simulink subsystem "throttleInput"  (R2022b)
settings: Solver=VariableStepAuto  StartTime=0.0  StopTime=10.0  RelTol=1e-3
libraries: throttleInput_lib x4, Raptor_lib x2
settings Model: Creator=serga  LastModifiedBy=serga

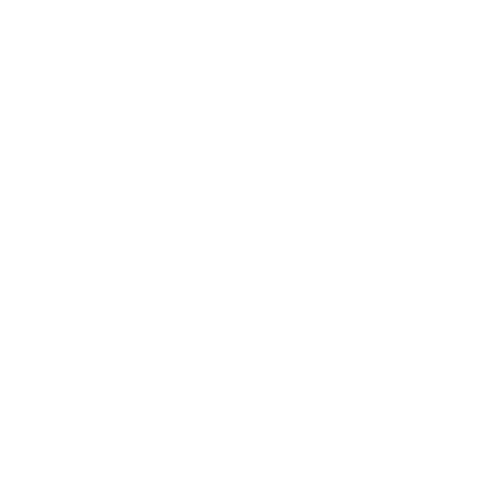
[thumbnail: Simulink's stored preview of the top-level diagram]
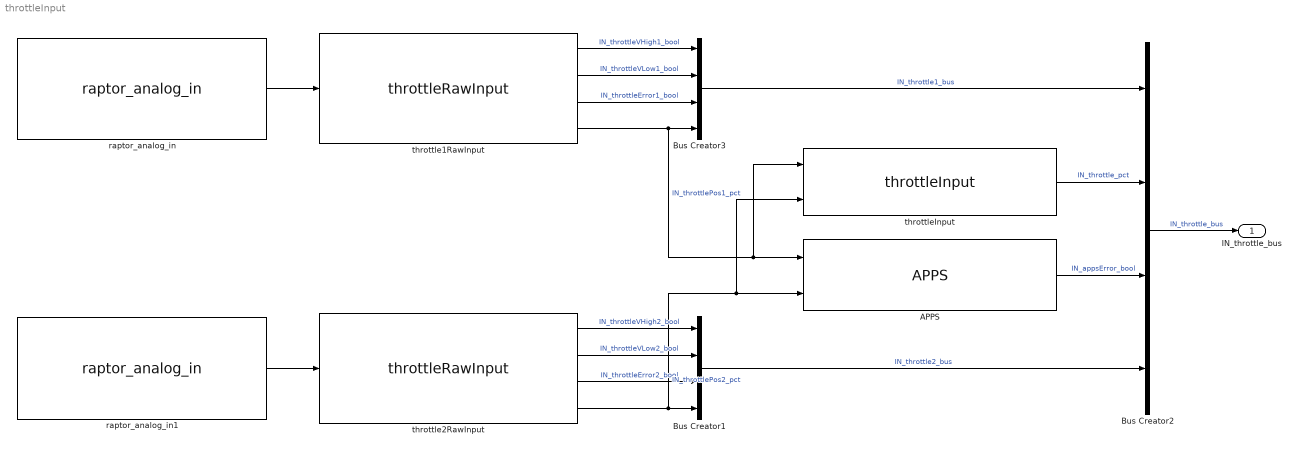
== system throttleInput ==
  APPS : throttleInput_lib/APPS  SystemSampleTime=-1  VariantActivationTime=update diagram  Latency=0  AutoFrameSizeCalculation=off
  Bus Creator1 : BusCreator  Inputs=4
  Bus Creator2 : BusCreator  Inputs=4
  Bus Creator3 : BusCreator  Inputs=4
  raptor_analog_in : Raptor_lib/Input & Output/raptor_analog_in  resourceValues=INPUT2|INPUT3|INPUT4|INPUT5|INPUT6|INPUT7|INPUT8|INPUT9|INPUT10|INPUT11|INPUT12|INPUT13|INPUT14|INPUT15|INPUT16|INPUT17|INPUT18|INPUT19|INPUT20|INPUT21|INPUT22|INPUT23|INPUT24|INPUT25|INPUT26|INPUT27|INPUT28|INPUT29|INPUT30|INPUT31|INPUT32|(None)  resource=INPUT3  rangeValues=0 - 5 V  range=0 - 5 V  filterrateValues=[]  filterrate='RAPTOR MASK DEFAULT'  resolutionValues=[]  resolution=[]  pullUDValues=2.15k PU  pullUD=2.15k PU
      settings: SourceProductName=Raptor
  raptor_analog_in1 : Raptor_lib/Input & Output/raptor_analog_in  resourceValues=INPUT2|INPUT3|INPUT4|INPUT5|INPUT6|INPUT7|INPUT8|INPUT9|INPUT10|INPUT11|INPUT12|INPUT13|INPUT14|INPUT15|INPUT16|INPUT17|INPUT18|INPUT19|INPUT20|INPUT21|INPUT22|INPUT23|INPUT24|INPUT25|INPUT26|INPUT27|INPUT28|INPUT29|INPUT30|INPUT31|INPUT32|(None)  resource=INPUT4  rangeValues=0 - 5 V  range=0 - 5 V  filterrateValues=[]  filterrate='RAPTOR MASK DEFAULT'  resolutionValues=[]  resolution=[]  pullUDValues=422k PD  pullUD=422k PD
      settings: SourceProductName=Raptor
  throttle1RawInput : throttleInput_lib/throttleRawInput  pos='1'
      settings: LibrarySourceBlock=throttleInput_lib/throttleInput
  throttle2RawInput : throttleInput_lib/throttleRawInput  pos='2'
      settings: LibrarySourceBlock=throttleInput_lib/throttleInput
  throttleInput : throttleInput_lib/throttleInput  SystemSampleTime=-1  VariantActivationTime=update diagram  Latency=0  AutoFrameSizeCalculation=off
  IN_throttle_bus : Outport  LockScale=on
  wires:
  raptor_analog_in1/1 -> throttle2RawInput/1
  raptor_analog_in/1 -> throttle1RawInput/1
  APPS/1 -> Bus Creator2/3  "IN_appsError_bool"
  throttle1RawInput/1 -> Bus Creator3/1  "IN_throttleVHigh1_bool"
  throttle1RawInput/3 -> Bus Creator3/3  "IN_throttleError1_bool"
  throttle1RawInput/2 -> Bus Creator3/2  "IN_throttleVLow1_bool"
  throttle1RawInput/4 -> Bus Creator3/4, APPS/1, throttleInput/1  "IN_throttlePos1_pct"
  throttle2RawInput/1 -> Bus Creator1/1  "IN_throttleVHigh2_bool"
  throttle2RawInput/2 -> Bus Creator1/2  "IN_throttleVLow2_bool"
  throttle2RawInput/3 -> Bus Creator1/3  "IN_throttleError2_bool"
  throttle2RawInput/4 -> Bus Creator1/4, APPS/2, throttleInput/2  "IN_throttlePos2_pct"
  Bus Creator3/1 -> Bus Creator2/1  "IN_throttle1_bus"
  Bus Creator1/1 -> Bus Creator2/4  "IN_throttle2_bus"
  Bus Creator2/1 -> IN_throttle_bus/1  "IN_throttle_bus"
  throttleInput/1 -> Bus Creator2/2  "IN_throttle_pct"
